simulink model "mass_damper_system"  (R2021b)
settings: Solver=VariableStepAuto  StartTime=0.0  StopTime=10  RelTol=1e-3
libraries: aerolibanimutils x1
settings Model: Creator=Joshua  LastModifiedBy=Joshua

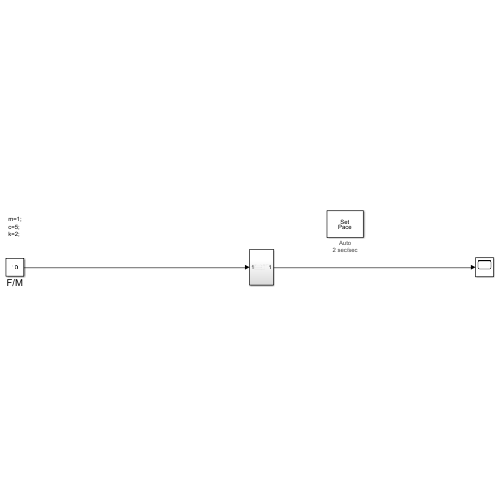
[thumbnail: Simulink's stored preview of the top-level diagram]
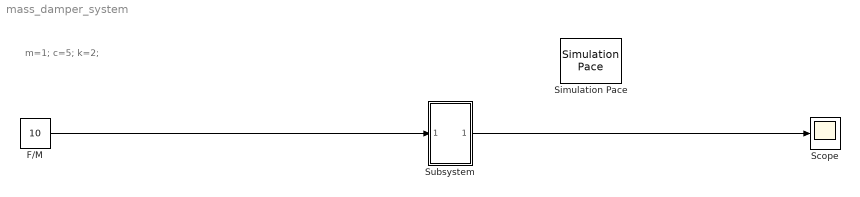
== system mass_damper_system ==
  note: m=1;
      | c=5;
      | k=2;
  F/M : Constant  Value=10
  Scope : Scope
  Simulation Pace : aerolibanimutils/Simulation Pace  SimulationPace=2  SleepMode=Auto  OutputPaceError=off  SampleTime=1/30
  Subsystem : Subsystem
  wires:
  F/M/1 -> Subsystem/1(In1)
  Subsystem/1(Out1) -> Scope/1

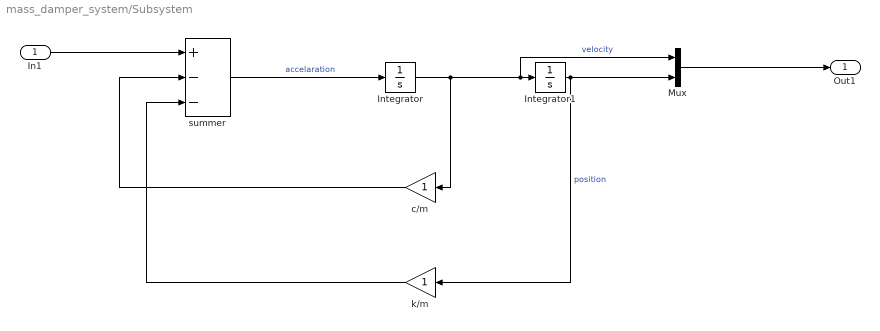
== system mass_damper_system/Subsystem ==
  In1 : Inport
  Integrator : Integrator
  Integrator1 : Integrator
  Mux : Mux  Inputs=2
  c/m : Gain
  k/m : Gain
  summer : Sum  Inputs=+--
  Out1 : Outport
  wires:
  summer/1 -> Integrator/1  "accelaration"
  Integrator/1 -> c/m/1, Mux/1, Integrator1/1  "velocity"
  c/m/1 -> summer/2
  Integrator1/1 -> k/m/1, Mux/2  "position"
  In1/1 -> summer/1
  k/m/1 -> summer/3
  Mux/1 -> Out1/1
